simulink model "sampleModel2029"  (R2023a)
settings: Solver=VariableStepAuto  StartTime=0.0  StopTime=10.0  RelTol=1e-3
libraries: hdlsllib x5, simulink x2
settings Model: Creator=user1  LastModifiedBy=user1

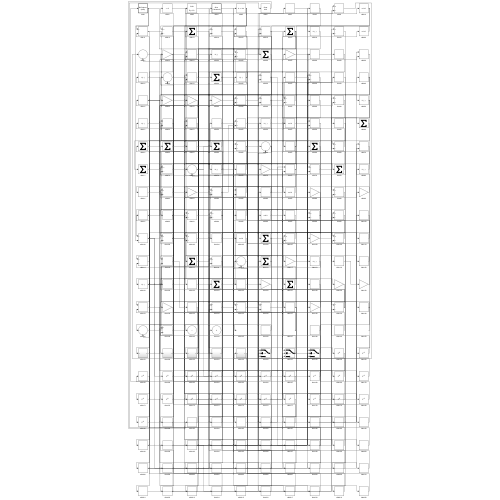
[thumbnail: Simulink's stored preview of the top-level diagram]
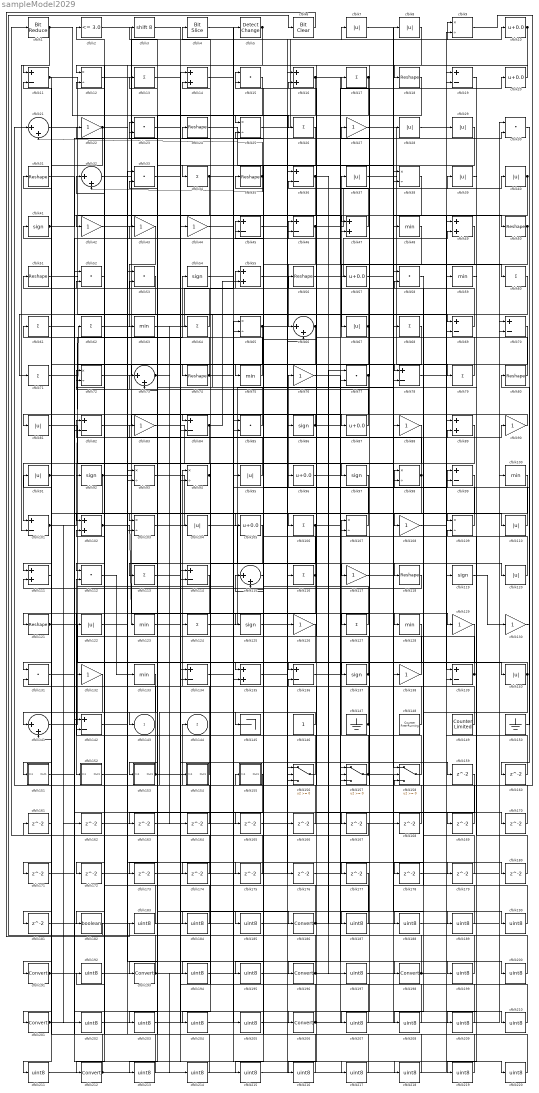
== system sampleModel2029 ==
  cfblk1 : hdlsllib/Logic and Bit Operations/Bit Reduce  mode=AND
  cfblk{10,20,57,87,96,105} (6 alike) : Bias  Bias=0.0  SaturateOnIntegerOverflow=off
  cfblk{48,59,63,75,100,123,128,133} (8 alike) : MinMax
  cfblk{11,19,36,45..46,69..70,78,82,84,99,101,114,134,136,139,142} (17 alike) : Sum  Inputs=+-
  cfblk{14,16,47,49,55,89,102,111,135} (9 alike) : Sum
  cfblk{9,12,25,38,65,72,93..94,98,103,107,109} (12 alike) : Product  Inputs=*/  RndMeth=Zero  SaturateOnIntegerOverflow=on
  cfblk{7..8,28..29,37,39..40,67,81,91,95,104,110,120,122,140} (16 alike) : Abs  SaturateOnIntegerOverflow=off
  cfblk{13,17,26,34,60..62,64,68,71,79,106,113,116,124,127} (16 alike) : Sum  Inputs=+
  cfblk{22,27,42..44,76,83,88,90,108,117,126,129..130,132,138} (16 alike) : Gain
  cfblk{15,23,30,33,52..53,58,77,85,112,131} (11 alike) : DotProduct  OutDataTypeStr=Inherit: Inherit via internal rule
  cfblk{21,32,66,73,115,141} (6 alike) : Sum  Inputs=|++
  cfblk{18,24,31,35,50..51,56,74,80,118,121} (11 alike) : Reshape
  cfblk{41,54,86,92,97,119,125,137} (8 alike) : Signum
  cfblk145 : Terminator
  cfblk146 : Constant  SampleTime=-1
  cfblk147 : Ground
  cfblk148 : hdlsllib/Sources/Counter Free-Running  NumBits=16  tsamp=-1
  cfblk149 : hdlsllib/Sources/Counter Limited  uplimit=7  tsamp=-1
  cfblk150 : Ground
  cfblk151 : Subsystem
      settings: LibrarySourceBlock=|
      | hdlsllib/Ports &
      | Subsystems/Subsystem
  cfblk152 : Subsystem
      settings: LibrarySourceBlock=|
      | hdlsllib/Ports &
      | Subsystems/Subsystem
  cfblk153 : Subsystem
      settings: LibrarySourceBlock=|
      | hdlsllib/Ports &
      | Subsystems/Subsystem
  cfblk154 : Subsystem
      settings: LibrarySourceBlock=|
      | hdlsllib/Ports &
      | Subsystems/Subsystem
  cfblk155 : Subsystem
      settings: LibrarySourceBlock=|
      | hdlsllib/Ports &
      | Subsystems/Subsystem
  cfblk156 : Switch  SaturateOnIntegerOverflow=off  InputSameDT=off
  cfblk157 : Switch  SaturateOnIntegerOverflow=off  InputSameDT=off
  cfblk158 : Switch  SaturateOnIntegerOverflow=off  InputSameDT=off
  cfblk{159..181} (23 alike) : Delay  SampleTime=1
  cfblk182 : DataTypeConversion  OutDataTypeStr=boolean  SaturateOnIntegerOverflow=off  RndMeth=Floor
  cfblk{183..185,187..190,192,194..195,197,199..200,202..205,207..211,213..220} (30 alike) : DataTypeConversion  OutDataTypeStr=uint8  SaturateOnIntegerOverflow=off  RndMeth=Floor
  cfblk{186,191,193,196,198,201,206,212} (8 alike) : DataTypeConversion  SaturateOnIntegerOverflow=off  RndMeth=Floor
  cfblk2 : hdlsllib/Logic and Bit Operations/Compare To Constant  relop=<=  const=3.0  OutDataTypeStr=boolean
  cfblk3 : ArithShift  BitShiftNumber=8
  cfblk4 : hdlsllib/Logic and Bit Operations/Bit Slice  lidx=7  ridx=0
  cfblk5 : simulink/Logic and Bit Operations/Detect Change  vinit=0  OutDataTypeStr=boolean
      settings: LibrarySourceBlock=|
      | hdlsllib/Logic and Bit
      | Operations/Detect
      | Change
  cfblk6 : simulink/Logic and Bit Operations/Bit Clear  iBit=0
      settings: LibrarySourceBlock=|
      | hdlsllib/Logic and Bit
      | Operations/Bit Clear
  cfblk143 : Outport  VectorParamsAs1DForOutWhenUnconnected=off
  cfblk144 : Outport  Port=2  VectorParamsAs1DForOutWhenUnconnected=off
  wires:
  cfblk84/1 -> cfblk101/1, cfblk55/2
  cfblk28/1 -> cfblk29/1
  cfblk27/1 -> cfblk79/1
  cfblk94/1 -> cfblk61/1, cfblk174/1
  cfblk59/1 -> cfblk71/1
  cfblk101/1 -> cfblk62/1, cfblk162/1, cfblk202/1
  cfblk142/1 -> cfblk198/1
  cfblk20/1 -> cfblk12/1
  cfblk49/1 -> cfblk66/1
  cfblk1/1 -> cfblk25/1, cfblk11/1, cfblk101/2
  cfblk103/1 -> cfblk110/1
  cfblk42/1 -> cfblk7/1
  cfblk2/1 -> cfblk74/1
  cfblk130/1 -> cfblk98/1
  cfblk66/1 -> cfblk34/1, cfblk73/2
  cfblk80/1 -> cfblk37/1
  cfblk11/1 -> cfblk89/1, cfblk151/1(In1)
  cfblk71/1 -> cfblk78/1
  cfblk36/1 -> cfblk135/2, cfblk82/2, cfblk197/1
  cfblk62/1 -> cfblk118/1
  cfblk34/1 -> cfblk42/1, cfblk120/1
  cfblk112/1 -> cfblk133/1
  cfblk15/1 -> cfblk143/1
  cfblk72/1 -> cfblk75/1
  cfblk69/1 -> cfblk4/1
  cfblk124/1 -> cfblk48/1
  cfblk109/1 -> cfblk56/1
  cfblk51/1 -> cfblk138/1
  cfblk114/1 -> cfblk201/1
  cfblk91/1 -> cfblk111/1, cfblk46/2
  cfblk61/1 -> cfblk46/1
  cfblk14/1 -> cfblk206/1
  cfblk87/1 -> cfblk73/1
  cfblk111/1 -> cfblk31/1
  cfblk41/1 -> cfblk106/1, cfblk47/2, cfblk30/2
  cfblk45/1 -> cfblk9/1
  cfblk77/1 -> cfblk17/1, cfblk93/2
  cfblk141/1 -> cfblk54/1
  cfblk85/1 -> cfblk51/1
  cfblk25/1 -> cfblk10/1
  cfblk82/1 -> cfblk87/1
  cfblk158/1 -> cfblk107/1
  cfblk24/1 -> cfblk158/1
  cfblk12/1 -> cfblk26/1
  cfblk10/1 -> cfblk18/1, cfblk97/1
  cfblk46/1 -> cfblk9/2, cfblk145/1
  cfblk9/1 -> cfblk144/1
  cfblk139/1 -> cfblk94/1, cfblk122/1
  cfblk63/1 -> cfblk5/1
  cfblk149/1 -> cfblk91/1
  cfblk128/1 -> cfblk152/1(In1)
  cfblk75/1 -> cfblk2/1
  cfblk116/1 -> cfblk45/1, cfblk132/1
  cfblk137/1 -> cfblk36/2, cfblk177/1, cfblk187/1
  cfblk37/1 -> cfblk59/1
  cfblk117/1 -> cfblk40/1
  cfblk40/1 -> cfblk112/1, cfblk103/1
  cfblk146/1 -> cfblk21/1
  cfblk38/1 -> cfblk193/1
  cfblk32/1 -> cfblk78/2
  cfblk138/1 -> cfblk3/1
  cfblk55/1 -> cfblk129/1
  cfblk133/1 -> cfblk141/1
  cfblk148/1 -> cfblk104/1
  cfblk7/1 -> cfblk50/1
  cfblk13/1 -> cfblk186/1
  cfblk156/1 -> cfblk112/2
  cfblk127/1 -> cfblk72/1
  cfblk53/1 -> cfblk131/1
  cfblk21/1 -> cfblk95/1
  cfblk26/1 -> cfblk153/1(In1)
  cfblk147/1 -> cfblk72/2, cfblk83/1
  cfblk125/1 -> cfblk99/1
  cfblk43/1 -> cfblk63/1
  cfblk73/1 -> cfblk64/1, cfblk164/1
  cfblk16/1 -> cfblk60/1, cfblk84/2
  cfblk67/1 -> cfblk27/1, cfblk105/1, cfblk57/1, cfblk182/1
  cfblk60/1 -> cfblk141/2
  cfblk4/1 -> cfblk136/1
  cfblk107/1 -> cfblk76/1
  cfblk140/1 -> cfblk137/1, cfblk178/1
  cfblk119/1 -> cfblk130/1
  cfblk150/1 -> cfblk80/1
  cfblk65/1 -> cfblk109/1, cfblk113/1
  cfblk79/1 -> cfblk15/1
  cfblk90/1 -> cfblk81/1
  cfblk57/1 -> cfblk28/1
  cfblk70/1 -> cfblk108/1
  cfblk50/1 -> cfblk69/1, cfblk69/2
  cfblk118/1 -> cfblk111/2
  cfblk106/1 -> cfblk125/1, cfblk190/1
  cfblk123/1 -> cfblk154/1(In1)
  cfblk154/1(Out1) -> cfblk124/1
  cfblk153/1(Out1) -> cfblk134/1, cfblk102/2
  cfblk102/1 -> cfblk123/1, cfblk89/2
  cfblk74/1 -> cfblk11/2, cfblk169/1
  cfblk35/1 -> cfblk15/2, cfblk21/2, cfblk32/2
  cfblk104/1 -> cfblk117/1
  cfblk110/1 -> cfblk45/2
  cfblk98/1 -> cfblk102/1, cfblk23/2
  cfblk113/1 -> cfblk44/1
  cfblk5/1 -> cfblk92/1, cfblk103/2, cfblk172/1
  cfblk92/1 -> cfblk128/1, cfblk171/1
  cfblk47/1 -> cfblk16/2
  cfblk68/1 -> cfblk191/1
  cfblk52/1 -> cfblk212/1
  cfblk108/1 -> cfblk90/1
  cfblk121/1 -> cfblk140/1, cfblk94/2, cfblk96/1
  cfblk157/1 -> cfblk24/1, cfblk189/1
  cfblk48/1 -> cfblk67/1
  cfblk78/1 -> cfblk119/1
  cfblk44/1 -> cfblk47/1
  cfblk22/1 -> cfblk121/1, cfblk180/1
  cfblk83/1 -> cfblk98/2
  cfblk8/1 -> cfblk196/1
  cfblk97/1 -> cfblk135/1
  cfblk120/1 -> cfblk55/1
  cfblk151/1(Out1) -> cfblk43/1
  cfblk64/1 -> cfblk23/1
  cfblk17/1 -> cfblk127/1, cfblk156/3, cfblk173/1
  cfblk93/1 -> cfblk139/1
  cfblk86/1 -> cfblk39/1, cfblk84/1
  cfblk56/1 -> cfblk49/2
  cfblk95/1 -> cfblk82/1
  cfblk81/1 -> cfblk157/1
  cfblk18/1 -> cfblk65/2
  cfblk136/1 -> cfblk20/1
  cfblk3/1 -> cfblk159/1
  cfblk30/1 -> cfblk160/1
  cfblk160/1 -> cfblk49/1
  cfblk162/1 -> cfblk134/2
  cfblk126/1 -> cfblk163/1
  cfblk163/1 -> cfblk66/2
  cfblk164/1 -> cfblk12/2
  cfblk23/1 -> cfblk165/1
  cfblk165/1 -> cfblk158/2
  cfblk166/1 -> cfblk25/2
  cfblk131/1 -> cfblk167/1
  cfblk167/1 -> cfblk1/1
  cfblk168/1 -> cfblk136/2
  cfblk169/1 -> cfblk16/1
  cfblk152/1(Out1) -> cfblk170/1
  cfblk170/1 -> cfblk107/2
  cfblk172/1 -> cfblk157/3
  cfblk174/1 -> cfblk32/1
  cfblk122/1 -> cfblk175/1
  cfblk175/1 -> cfblk93/1
  cfblk135/1 -> cfblk176/1
  cfblk176/1 -> cfblk157/2
  cfblk178/1 -> cfblk70/2
  cfblk96/1 -> cfblk179/1
  cfblk179/1 -> cfblk158/3
  cfblk180/1 -> cfblk109/2
  cfblk132/1 -> cfblk181/1
  cfblk181/1 -> cfblk65/1
  cfblk182/1 -> cfblk6/1
  cfblk6/1 -> cfblk183/1
  cfblk183/1 -> cfblk22/1
  cfblk100/1 -> cfblk184/1
  cfblk184/1 -> cfblk53/1
  cfblk89/1 -> cfblk185/1
  cfblk185/1 -> cfblk100/1
  cfblk186/1 -> cfblk53/2, cfblk77/1
  cfblk187/1 -> cfblk13/1
  cfblk58/1 -> cfblk188/1
  cfblk188/1 -> cfblk30/1
  cfblk189/1 -> cfblk58/1
  cfblk190/1 -> cfblk58/2
  cfblk191/1 -> cfblk116/1, cfblk41/1
  cfblk192/1 -> cfblk68/1
  cfblk193/1 -> cfblk168/1, cfblk166/1, cfblk131/2, cfblk214/1
  cfblk105/1 -> cfblk194/1
  cfblk194/1 -> cfblk38/1
  cfblk29/1 -> cfblk195/1
  cfblk195/1 -> cfblk38/2
  cfblk196/1 -> cfblk139/2, cfblk156/1
  cfblk197/1 -> cfblk8/1
  cfblk198/1 -> cfblk36/1, cfblk35/1
  cfblk76/1 -> cfblk199/1
  cfblk199/1 -> cfblk142/1
  cfblk173/1 -> cfblk200/1
  cfblk200/1 -> cfblk142/2
  cfblk201/1 -> cfblk77/2, cfblk70/1, cfblk126/1
  cfblk202/1 -> cfblk114/1
  cfblk177/1 -> cfblk203/1
  cfblk203/1 -> cfblk114/2
  cfblk88/1 -> cfblk204/1
  cfblk204/1 -> cfblk85/2
  cfblk54/1 -> cfblk205/1
  cfblk205/1 -> cfblk88/1
  cfblk206/1 -> cfblk156/2, cfblk85/1
  cfblk99/1 -> cfblk207/1
  cfblk207/1 -> cfblk14/1
  cfblk129/1 -> cfblk208/1
  cfblk208/1 -> cfblk14/2
  cfblk19/1 -> cfblk209/1
  cfblk209/1 -> cfblk155/1(In1)
  cfblk31/1 -> cfblk210/1
  cfblk210/1 -> cfblk19/1
  cfblk161/1 -> cfblk211/1
  cfblk211/1 -> cfblk19/2
  cfblk212/1 -> cfblk161/1, cfblk99/2
  cfblk155/1(Out1) -> cfblk213/1
  cfblk213/1 -> cfblk52/1
  cfblk214/1 -> cfblk52/2
  cfblk115/1 -> cfblk215/1
  cfblk215/1 -> cfblk86/1
  cfblk159/1 -> cfblk216/1
  cfblk216/1 -> cfblk115/1
  cfblk134/1 -> cfblk217/1
  cfblk217/1 -> cfblk115/2
  cfblk33/1 -> cfblk218/1
  cfblk218/1 -> cfblk192/1
  cfblk39/1 -> cfblk219/1
  cfblk219/1 -> cfblk33/1
  cfblk171/1 -> cfblk220/1
  cfblk220/1 -> cfblk33/2

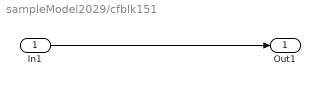
== system sampleModel2029/cfblk151 ==
  In1 : Inport
  Out1 : Outport
  wires:
  In1/1 -> Out1/1

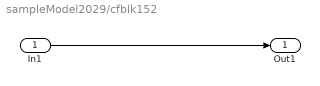
== system sampleModel2029/cfblk152 ==
  In1 : Inport
  Out1 : Outport
  wires:
  In1/1 -> Out1/1

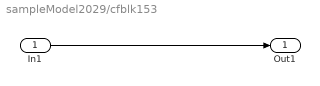
== system sampleModel2029/cfblk153 ==
  In1 : Inport
  Out1 : Outport
  wires:
  In1/1 -> Out1/1

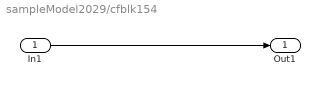
== system sampleModel2029/cfblk154 ==
  In1 : Inport
  Out1 : Outport
  wires:
  In1/1 -> Out1/1

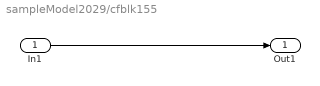
== system sampleModel2029/cfblk155 ==
  In1 : Inport
  Out1 : Outport
  wires:
  In1/1 -> Out1/1
